simulink model "power_busbar"  (Simulink 6.0)
settings: Solver=ode15s  SolverMode=SingleTasking  StartTime=0.0  StopTime=10.0  RelTol=1e-3  AbsTol=1e-6
libraries: powerlib x9
settings Model: Creator=patrice  LastModifiedBy=batserve  ExtModeTrigMode=oneshot  ExtModeArmWhenConnect=off  ExtModeAutoUpdateStatusClock=off
settings DataIOCC: LimitDataPoints=off  SignalLoggingName=sigsOut
settings OptimizationCC: BooleanDataType=off
settings DebuggingCC: SolverPrmCheckMsg=none
settings HardwareCC: TargetUnknown=on
settings RTWCC: TemplateMakefile=grt_unix.tmf

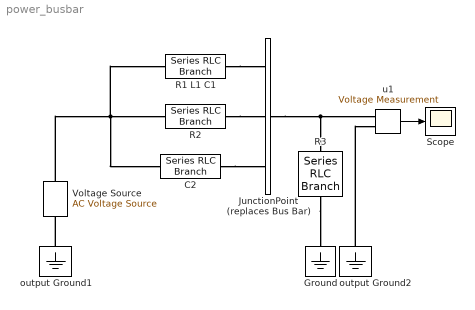
== system power_busbar ==
  C2 : powerlib/Elements/Series RLC Branch  PhysicalDomain=powersysdomain  SubClassName=unknown  PortType=p1  LConnTagsString=__new0  RConnTagsString=__new0  Resistance=0  Inductance=0  Capacitance=1  Measurements=None
  Ground : powerlib/Elements/Ground  Orientation=down  PhysicalDomain=powersysdomain  SubClassName=unknown  PortType=p1  LConnTagsString=a
  "JunctionPoint (replaces Bus Bar) " : PMComponent  Tag=PoWeRsYsTeMbLoCk  PhysicalDomain=powersysdomain  LeftPortType=p1  RightPortType=p1  LConnTagsString=I1|I2|I3  RConnTagsString=O1  mask(JunctionPoint){entrees=3, sorties=1}
      mask prompts: entrees "inputs"; sorties "outputs"
      mask help: This block is used to replace the Bus Bar block from powerlib2. This block was generated by the psbupdate function. With SimPowerSystems, this block is not required. You should considere deleting this block and reconnect the lines together.
      mask init:
      | inputtags = cell(1,entrees);
      | 
      | for i=1:entrees
      | 
      | 	inputtags{i} = ['I',num2str(i)];
      | 
      | end
      | 
      | outputtags = cell(1,sorties);
      | 
      | for i=1:sorties
      | 
      | 	outputtags{i} = ['O',num2str(i)];
      | 
      | end
      | 
      | set_param(gcbh,'LConnTags',inputtags);
      | 
      | set_param(gcbh,'RConnTags',outputtags);
      mask Display:
      | color('red');
      | 
      | plot([0,100],[0,100])
      | 
      | plot([0,100],[100,0])
  R1 L1 C1 : powerlib/Elements/Series RLC Branch  PhysicalDomain=powersysdomain  SubClassName=unknown  PortType=p1  LConnTagsString=__new0  RConnTagsString=__new0  Resistance=1  Inductance=1e-03  Capacitance=1e-06  Measurements=None
  R2 : powerlib/Elements/Series RLC Branch  PhysicalDomain=powersysdomain  SubClassName=unknown  PortType=p1  LConnTagsString=__new0  RConnTagsString=__new0  Resistance=1  Inductance=0  Capacitance=inf  Measurements=None
  R3 : powerlib/Elements/Series RLC Branch  Orientation=down  PhysicalDomain=powersysdomain  SubClassName=unknown  PortType=p1  LConnTagsString=__new0  RConnTagsString=__new0  Resistance=1  Inductance=0  Capacitance=inf  Measurements=None
  Scope : Scope
      settings: TickLabels=on  TimeRange=0.1  YMin=-50  YMax=50  DataFormat=Array
  Voltage Source : powerlib/Electrical Sources/AC Voltage Source  Description=source block  Orientation=up  Amplitude=50  Phase=0  Frequency=60  SampleTime=0  Measurements=None
      settings: AttributesFormatString=\n
  output Ground1 : powerlib/Elements/Ground  Orientation=down  PhysicalDomain=powersysdomain  SubClassName=unknown  PortType=p1  LConnTagsString=a
  output Ground2 : powerlib/Elements/Ground  Orientation=down  PhysicalDomain=powersysdomain  SubClassName=unknown  PortType=p1  LConnTagsString=a
  u1 : powerlib/Measurements/Voltage Measurement  Tag=PoWeRsYsTeMmEaSuReMeNt  PhasorSimulation=off  OutputType=Magnitude  PSBequivalent=0
  wires:
  u1/1 -> Scope/1
  connections:
  R3/RConn1 -- Ground/LConn1
  "JunctionPoint (replaces Bus Bar) "/RConn1 -- R3/LConn1 -- u1/LConn1
  output Ground2/LConn1 -- u1/LConn2
  output Ground1/LConn1 -- Voltage Source/LConn1
  R1 L1 C1/RConn1 -- "JunctionPoint (replaces Bus Bar) "/LConn1
  R2/RConn1 -- "JunctionPoint (replaces Bus Bar) "/LConn2
  C2/RConn1 -- "JunctionPoint (replaces Bus Bar) "/LConn3
  Voltage Source/RConn1 -- R2/LConn1 -- R1 L1 C1/LConn1 -- C2/LConn1
